simulink model "vehicle_slip_regulation"  (R2018a)
settings: Solver=ode4  StartTime=0.0  StopTime=300  FixedStep=0.001  RelTol=1e-3
values from neighbouring files (symbols this model uses):
  B0 = 2.5    [init_params.m]
  Is = 0.2    [init_params.m]
  m = 100    [init_params.m]
  MFC1 = [9.5 1.9 1.14  0.75]    [init_params.m]
  MFC2 = [2.5 1.8 1 0.2]    [init_params.m]
  MFC3 = [1.5 1.8 0.4 0.2]    [init_params.m]
  N = 500    [init_params.m]
  r = 0.2    [init_params.m]
  v0 = 1    [init_params.m]
libraries: simulink x1
settings Model: Creator=obrusvit  LastModifiedBy=obrusvit

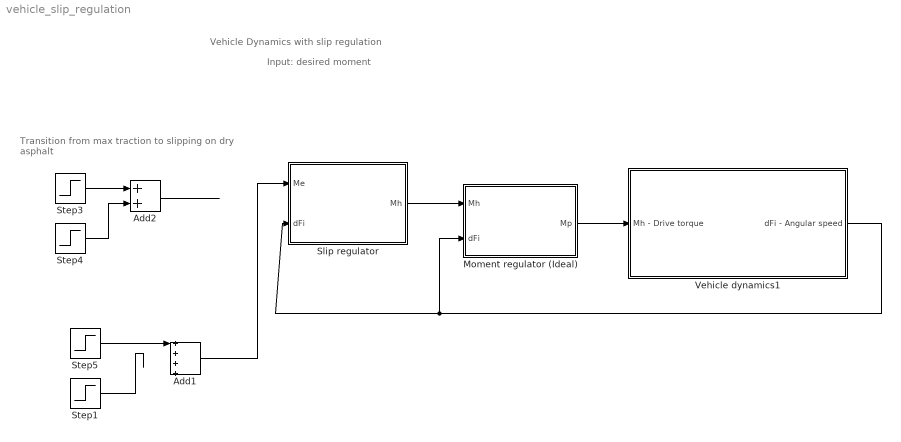
== system vehicle_slip_regulation ==
  note: Input: desired moment
  note: Vehicle Dynamics with slip regulation
  note: Transition from max traction to slipping
      | on dry asphalt
  Add1 : Sum  Inputs=++++
  Add2 : Sum
  Moment regulator (Ideal) : Subsystem
  Slip regulator : Subsystem
  Step1 : Step  Time=75  After=-90  SampleTime=0
  Step3 : Step  Time=10  After=110  SampleTime=0
  Step4 : Step  Time=50  After=5  SampleTime=0
  Step5 : Step  Time=5  After=110  SampleTime=0
  Vehicle dynamics1 : Subsystem
  wires:
  Moment regulator (Ideal)/1("Mp ") -> Vehicle dynamics1/1(Mh - Drive torque)
  Slip regulator/1("Mh ") -> Moment regulator (Ideal)/1(Mh)
  Vehicle dynamics1/1(dFi - Angular speed) -> Moment regulator (Ideal)/2(dFi), Slip regulator/2(dFi)
  Add2/1 -> ?
  Step4/1 -> Add2/2
  Step3/1 -> Add2/1
  Step5/1 -> Add1/1
  Add1/1 -> Slip regulator/1(Me)
  Step1/1 -> ?
  ? -> Add1/3

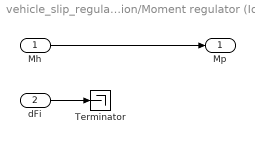
== system vehicle_slip_regulation/Moment regulator (Ideal) ==
  Mh : Inport
  dFi : Inport  Port=2
  Terminator : Terminator
  "Mp " : Outport
  wires:
  Mh/1 -> "Mp "/1
  dFi/1 -> Terminator/1

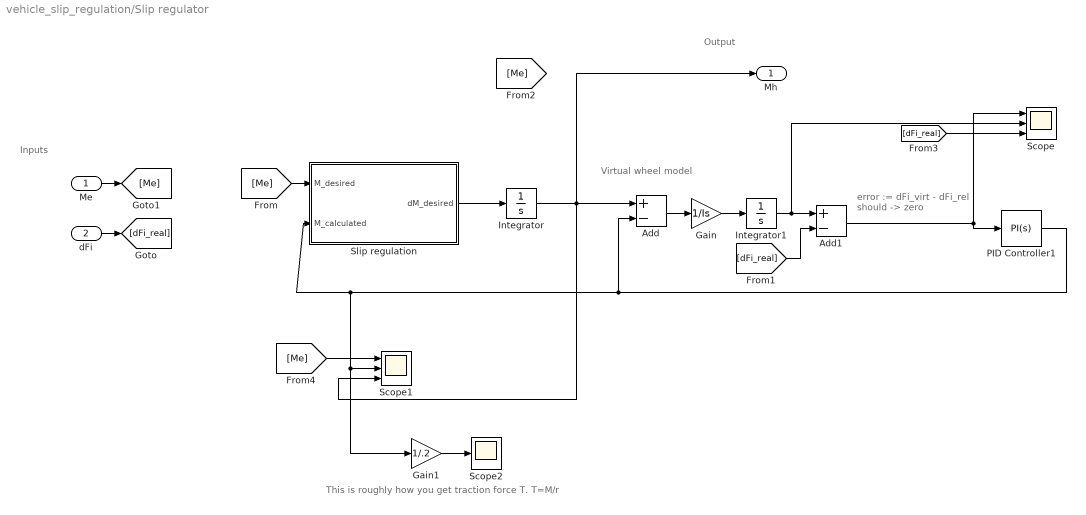
== system vehicle_slip_regulation/Slip regulator ==
  note: This is roughly how you get traction force T. T=M/r
  note: error := dFi_virt - dFi_rel
      | should -> zero
  note: Virtual wheel model
  note: Output
  note: Inputs
  Me : Inport
  dFi : Inport  Port=2
  Add : Sum  Inputs=+-
  Add1 : Sum  Inputs=+-
  Gain : Gain  Gain=1/Is
  Gain1 : Gain  Gain=1/.2
  Integrator : Integrator
  Integrator1 : Integrator
  PID Controller1 : simulink/Continuous/PID Controller  Controller=PI  TimeDomain=Continuous-time  SampleTime=-1  IntegratorMethod=Forward Euler  FilterMethod=Forward Euler  Form=Parallel  UseFilter=on  ControllerParametersSource=internal  P=15  I=20  D=0  N=100  InitialConditionSource=internal  InitialConditionForIntegrator=0  InitialConditionForFilter=0  ExternalReset=none  LimitOutput=on  UpperSaturationLimit=inf  LowerSaturationLimit=0  LinearizeAsGain=on  AntiWindupMode=none  Kb=1  TrackingMode=off  Kt=1  PParamMin=[]  PParamMax=[]  IParamMin=[]  IParamMax=[]  DParamMin=[]  DParamMax=[]  NParamMin=[]  NParamMax=[]  KbParamMin=[]  KbParamMax=[]  KtParamMin=[]  KtParamMax=[]  POutMin=[]  POutMax=[]  IOutMin=[]  IOutMax=[]  DOutMin=[]  DOutMax=[]  NOutMin=[]  NOutMax=[]  KbOutMin=[]  KbOutMax=[]  KtOutMin=[]  KtOutMax=[]  IntegratorOutMin=[]  IntegratorOutMax=[]  FilterOutMin=[]  FilterOutMax=[]  SumOutMin=[]  SumOutMax=[]  SumI1OutMin=[]  SumI1OutMax=[]  SumI2OutMin=[]  SumI2OutMax=[]  SumI3OutMin=[]  SumI3OutMax=[]  SumDOutMin=[]  SumDOutMax=[]  SaturationOutMin=[]  SaturationOutMax=[]  IntegratorContinuousStateAttributes=''  IntegratorStateMustResolveToSignalObject=off  IntegratorRTWStateStorageClass=Auto  FilterContinuousStateAttributes=''  FilterStateMustResolveToSignalObject=off  FilterRTWStateStorageClass=Auto  DifferentiatorICPrevScaledInput=0  DifferentiatorOutMin=[]  DifferentiatorOutMax=[]  FilterDiffOutCoefMin=[]  FilterDiffOutCoefMax=[]  SumDenOutMin=[]  SumDenOutMax=[]  SumNumOutMin=[]  SumNumOutMax=[]  ReciprocalOutMin=[]  ReciprocalOutMax=[]  DivideOutMin=[]  DivideOutMax=[]  TunerSelectOption=Transfer Function Based (PID Tuner App)
  Scope : Scope  NumInputPorts=3
  Scope1 : Scope  NumInputPorts=3
  Scope2 : Scope
  Slip regulation : MATLAB Function  TreatAsAtomicUnit=on
  "Mh " : Outport
  wires:
  dFi/1 -> [dFi_real]
  Me/1 -> [Me]
  [Me] -> Slip regulation/1(M_desired)
  Slip regulation/1(dM_desired) -> Integrator/1
  Add/1 -> Gain/1
  Gain/1 -> Integrator1/1
  [dFi_real] -> Add1/2
  Add1/1 -> PID Controller1/1, Scope/1
  Integrator/1 -> Scope1/3, "Mh "/1, Add/1
  Integrator1/1 -> Scope/2, Add1/1
  [dFi_real] -> Scope/3
  PID Controller1/1 -> Scope1/2, Gain1/1, Slip regulation/2(M_calculated), Add/2
  [Me] -> Scope1/1
  Gain1/1 -> Scope2/1

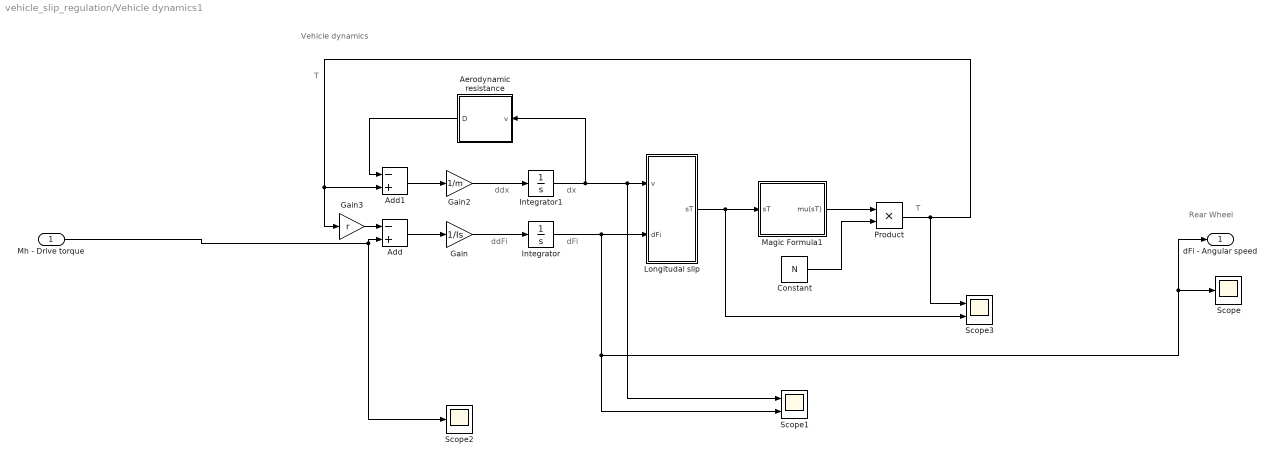
== system vehicle_slip_regulation/Vehicle dynamics1 ==
  note: Vehicle dynamics
  note: Rear Wheel
  note: T
  note: ddx
  note: dx
  note: ddFi
  note: T
  note: dFi
  Mh - Drive torque : Inport
  Add : Sum  Inputs=-+
  Add1 : Sum  Inputs=-+
  "Aerodynamic resistance " : Subsystem
  Constant : Constant  Value=N
  Gain : Gain  Gain=1/Is
  Gain2 : Gain  Gain=1/m
  Gain3 : Gain  Gain=r
  Integrator : Integrator  InitialCondition=v0/r
  Integrator1 : Integrator  InitialCondition=v0
  Longitudal slip : Subsystem
  Magic Formula1 : Subsystem
  Product : Product
  Scope : Scope
  Scope1 : Scope  NumInputPorts=2
  Scope2 : Scope
  Scope3 : Scope  NumInputPorts=2
  dFi - Angular speed : Outport
  wires:
  Longitudal slip/1(sT) -> Magic Formula1/1(sT), Scope3/2
  Add1/1 -> Gain2/1
  Product/1 -> Gain3/1, Add1/2, Scope3/1
  Integrator1/1 -> "Aerodynamic resistance "/1(v), Scope1/1, Longitudal slip/1(v)
  "Aerodynamic resistance "/1("D ") -> Add1/1
  Gain3/1 -> Add/1
  Magic Formula1/1(mu(sT)) -> Product/1
  Gain/1 -> Integrator/1
  Add/1 -> Gain/1
  Mh - Drive torque/1 -> Scope2/1, Add/2
  Constant/1 -> Product/2
  Integrator/1 -> Scope1/2, dFi - Angular speed/1, Scope/1, Longitudal slip/2(dFi)
  Gain2/1 -> Integrator1/1

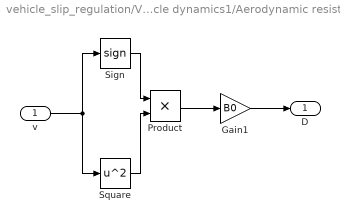
== system vehicle_slip_regulation/Vehicle dynamics1/Aerodynamic resistance  ==
  v : Inport
  Gain1 : Gain  Gain=B0
  Product : Product
  Sign : Signum
  Square : Math  Operator=square  SaturateOnIntegerOverflow=on
  "D " : Outport
  wires:
  v/1 -> Sign/1, Square/1
  Square/1 -> Product/2
  Sign/1 -> Product/1
  Gain1/1 -> "D "/1
  Product/1 -> Gain1/1

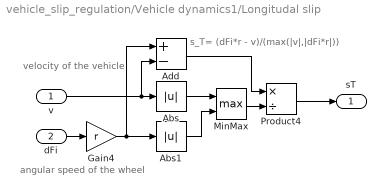
== system vehicle_slip_regulation/Vehicle dynamics1/Longitudal slip ==
  note: s_T= (dFi*r - v)/(max(|v|,|dFi*r|))
  note: angular speed
      | of the wheel
  note: velocity
      | of the vehicle
  v : Inport
  dFi : Inport  Port=2
  Abs : Abs
  Abs1 : Abs
  Add : Sum  Inputs=+-
  Gain4 : Gain  Gain=r
  MinMax : MinMax  Function=max  Inputs=2
  Product4 : Product  Inputs=*/  RndMeth=Zero
  sT : Outport
  wires:
  Product4/1 -> sT/1
  Add/1 -> Product4/1
  Abs1/1 -> MinMax/2
  Abs/1 -> MinMax/1
  MinMax/1 -> Product4/2
  Gain4/1 -> Add/1, Abs1/1
  dFi/1 -> Gain4/1
  v/1 -> Add/2, Abs/1

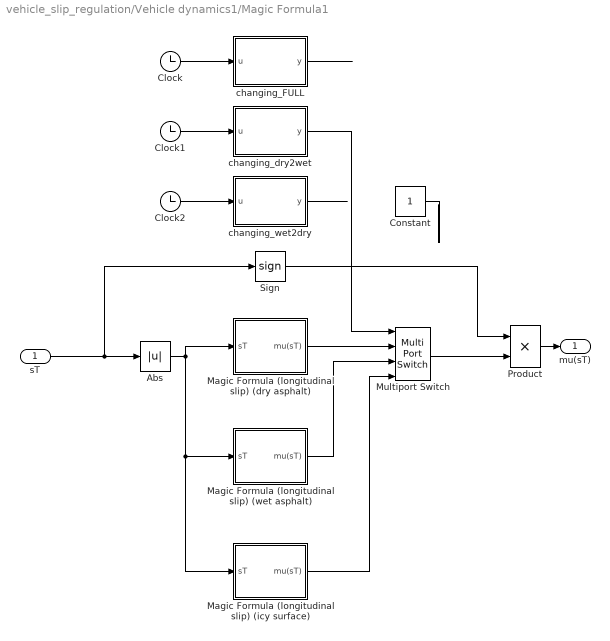
== system vehicle_slip_regulation/Vehicle dynamics1/Magic Formula1 ==
  sT : Inport
  Abs : Abs
  Clock : Clock
  Clock1 : Clock
  Clock2 : Clock
  Constant : Constant
  Magic Formula (longitudinal slip) (dry asphalt) : Subsystem
  Magic Formula (longitudinal slip) (icy surface) : Subsystem
  Magic Formula (longitudinal slip) (wet asphalt) : Subsystem
  Multiport Switch : MultiPortSwitch
  Product : Product
  Sign : Signum
  changing_FULL : MATLAB Function  TreatAsAtomicUnit=on
  changing_dry2wet : MATLAB Function  TreatAsAtomicUnit=on
  "changing_wet2dry " : MATLAB Function  TreatAsAtomicUnit=on
  mu(sT) : Outport
  wires:
  Abs/1 -> Magic Formula (longitudinal slip) (icy surface)/1(sT), Magic Formula (longitudinal slip) (wet asphalt)/1(sT), Magic Formula (longitudinal slip) (dry asphalt)/1(sT)
  Magic Formula (longitudinal slip) (dry asphalt)/1(mu(sT)) -> Multiport Switch/2
  Product/1 -> mu(sT)/1
  Sign/1 -> Product/1
  sT/1 -> Sign/1, Abs/1
  Magic Formula (longitudinal slip) (wet asphalt)/1(mu(sT)) -> Multiport Switch/3
  Multiport Switch/1 -> Product/2
  Magic Formula (longitudinal slip) (icy surface)/1(mu(sT)) -> Multiport Switch/4
  Clock/1 -> changing_FULL/1(u)
  changing_FULL/1(y) -> ?
  Constant/1 -> ?
  Clock1/1 -> changing_dry2wet/1(u)
  "changing_wet2dry "/1(y) -> ?
  Clock2/1 -> "changing_wet2dry "/1(u)
  changing_dry2wet/1(y) -> Multiport Switch/1

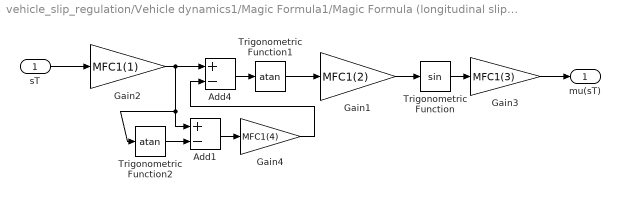
== system vehicle_slip_regulation/Vehicle dynamics1/Magic Formula1/Magic Formula (longitudinal slip) (dry asphalt) ==
  sT : Inport
  Add1 : Sum  Inputs=+-
  Add4 : Sum  Inputs=+-
  Gain1 : Gain  Gain=MFC1(2)
  Gain2 : Gain  Gain=MFC1(1)
  Gain3 : Gain  Gain=MFC1(3)
  Gain4 : Gain  Gain=MFC1(4)
  Trigonometric Function : Trigonometry
  Trigonometric Function1 : Trigonometry  Operator=atan
  Trigonometric Function2 : Trigonometry  Operator=atan
  mu(sT) : Outport
  wires:
  Gain3/1 -> mu(sT)/1
  sT/1 -> Gain2/1
  Add4/1 -> Trigonometric Function1/1
  Gain4/1 -> Add4/2
  Add1/1 -> Gain4/1
  Trigonometric Function2/1 -> Add1/2
  Gain2/1 -> Trigonometric Function2/1, Add1/1, Add4/1
  Trigonometric Function1/1 -> Gain1/1
  Gain1/1 -> Trigonometric Function/1
  Trigonometric Function/1 -> Gain3/1

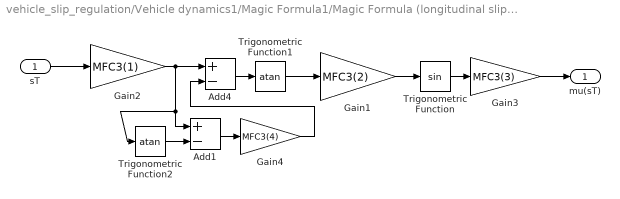
== system vehicle_slip_regulation/Vehicle dynamics1/Magic Formula1/Magic Formula (longitudinal slip) (icy surface) ==
  sT : Inport
  Add1 : Sum  Inputs=+-
  Add4 : Sum  Inputs=+-
  Gain1 : Gain  Gain=MFC3(2)
  Gain2 : Gain  Gain=MFC3(1)
  Gain3 : Gain  Gain=MFC3(3)
  Gain4 : Gain  Gain=MFC3(4)
  Trigonometric Function : Trigonometry
  Trigonometric Function1 : Trigonometry  Operator=atan
  Trigonometric Function2 : Trigonometry  Operator=atan
  mu(sT) : Outport
  wires:
  Gain3/1 -> mu(sT)/1
  sT/1 -> Gain2/1
  Add4/1 -> Trigonometric Function1/1
  Gain4/1 -> Add4/2
  Add1/1 -> Gain4/1
  Trigonometric Function2/1 -> Add1/2
  Gain2/1 -> Trigonometric Function2/1, Add1/1, Add4/1
  Trigonometric Function1/1 -> Gain1/1
  Gain1/1 -> Trigonometric Function/1
  Trigonometric Function/1 -> Gain3/1

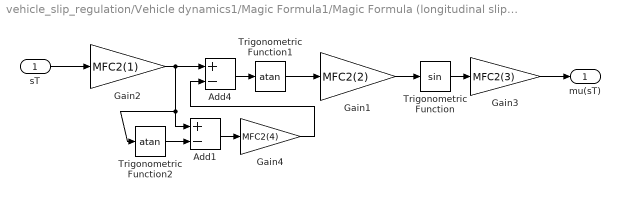
== system vehicle_slip_regulation/Vehicle dynamics1/Magic Formula1/Magic Formula (longitudinal slip) (wet asphalt) ==
  sT : Inport
  Add1 : Sum  Inputs=+-
  Add4 : Sum  Inputs=+-
  Gain1 : Gain  Gain=MFC2(2)
  Gain2 : Gain  Gain=MFC2(1)
  Gain3 : Gain  Gain=MFC2(3)
  Gain4 : Gain  Gain=MFC2(4)
  Trigonometric Function : Trigonometry
  Trigonometric Function1 : Trigonometry  Operator=atan
  Trigonometric Function2 : Trigonometry  Operator=atan
  mu(sT) : Outport
  wires:
  Gain3/1 -> mu(sT)/1
  sT/1 -> Gain2/1
  Add4/1 -> Trigonometric Function1/1
  Gain4/1 -> Add4/2
  Add1/1 -> Gain4/1
  Trigonometric Function2/1 -> Add1/2
  Gain2/1 -> Trigonometric Function2/1, Add1/1, Add4/1
  Trigonometric Function1/1 -> Gain1/1
  Gain1/1 -> Trigonometric Function/1
  Trigonometric Function/1 -> Gain3/1

== matlab function vehicle_slip_regulation/Vehicle dynamics1/Magic Formula1/changing_FULL ==
  data: u input; y output
function y = fcn(u)
if u <= 20
    y = 1;
elseif u <= 40
    y = 2;
elseif u <= 60
    y = 3;
elseif u <= 80
    y = 2;
else
    y = 1;
end
end

== matlab function vehicle_slip_regulation/Slip regulator/Slip regulation ==
  settings: updateMethod=DISCRETE
  data: M_desired input; dM_desired output; M_calculated input
function dM_desired = fcn(M_desired, M_calculated)

%% Vars management
persistent directionToGo;
persistent M_calculated_prev;
ERR_TOLERABLE = 1;
dM_INCREMENT = 5;

if isempty(directionToGo)
  directionToGo = 1;
end

if isempty(M_calculated_prev)
    % first time initialization of variable
    M_calculated_prev = 0;
end

%% Main algo
diff = M_desired - M_calculated;

if abs(diff) <= ERR_TOLERABLE
    directionToGo = 0;
    dM_desired = 0;
elseif diff > 0

    if ((directionToGo == 1) && (M_calculated_prev < M_calculated))
        % all right we can increase further
        directionToGo = 1;
        dM_desired = dM_INCREMENT;  
    elseif ((directionToGo == 1) && (M_calculated_prev > M_calculated))
        % we probably overshoot the maximum and we should decrement now
        directionToGo = -1;
        dM_desired = -dM_INCREMENT;
    
    elseif ((directionToGo == -1) && (M_calculated_prev > M_calculated))
        directionToGo = -1;
        dM_desired = -dM_INCREMENT;
    elseif ((directionToGo == -1) && (M_calculated_prev < M_calculated))
        % We need to go up again
        directionToGo = 1;
        dM_desired = dM_INCREMENT;
    else
        directionToGo = 1;
        dM_desired = dM_INCREMENT;
    end
        
else 
    directionToGo = -1;
    dM_desired = -dM_INCREMENT;
end

M_calculated_prev = M_calculated;
end

== matlab function vehicle_slip_regulation/Vehicle dynamics1/Magic Formula1/changing_dry2wet ==
  data: u input; y output
function y = fcn(u)
if u <= 150
    y = 3;
else
    y = 1;
end
end

== matlab function vehicle_slip_regulation/Vehicle dynamics1/Magic Formula1/changing_wet2dry  ==
  data: u input; y output
function y = fcn(u)
if u <= 150
    y = 2;
else
    y = 1;
end
end
